simulink model "lab5"  (R2014b)
settings: Solver=ode45  SolverMode=SingleTasking  StartTime=0.0  StopTime=10  RelTol=1e-3
libraries: truetime x1
settings Model: Creator=peterfj  LastModifiedBy=andfro
settings OptimizationCC: BlockReduction=off  BooleanDataType=off  UseDivisionForNetSlopeComputation=off  SimCompilerOptimization=off
settings DebuggingCC: SaveWithParameterizedLinksMsg=none  UnderspecifiedInitializationDetection=Classic  MergeDetectMultiDrivingBlocksExec=none  SignalResolutionControl=TryResolveAllWithWarning  SolverPrmCheckMsg=none  FrameProcessingCompatibilityMsg=error  AllowSymbolicDim=off
settings HardwareCC: TargetUnknown=on
settings RTWCC: RTWCompilerOptimization=off
settings ConfigComp: CovMetricSettings=dw  CovHtmlReporting=on  CovSaveCumulativeToWorkspaceVar=on  CovSaveSingleToWorkspaceVar=on  CovModelRefEnable=Off  CovExternalEMLEnable=off  CovSFcnEnable=off

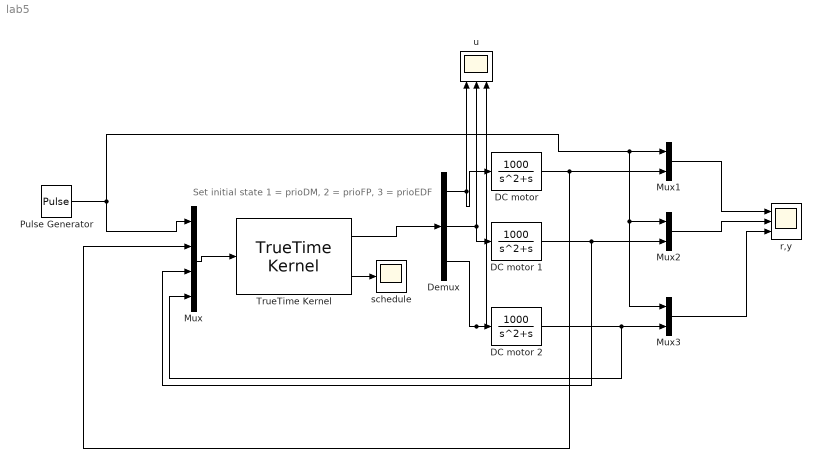
== system lab5 ==
  note: Set initial state 1 = prioDM, 2 = prioFP, 3 = prioEDF
  "DC motor " : TransferFcn  Numerator=[1000]  Denominator=[1 1 0]
  DC motor 1 : TransferFcn  Numerator=[1000]  Denominator=[1 1 0]
  DC motor 2 : TransferFcn  Numerator=[1000]  Denominator=[1 1 0]
  Demux : Demux  Outputs=3
  Mux : Mux
  Mux1 : Mux  Inputs=2
  Mux2 : Mux  Inputs=2
  Mux3 : Mux  Inputs=2
  Pulse Generator : DiscretePulseGenerator  PulseType=Time based  Amplitude=2  Period=1  PulseWidth=50  PhaseDelay=0.1  SampleTime=0.005
  TrueTime Kernel : truetime/TrueTime Kernel  sfun=node_init_3  args=1  ninputsoutputs=[4 3]  ntriggers=0  trigtype=falling  nwnodenbr=[]  clockoffsetdrift=[0 0]  schedoutput=on  battery=off  poweroutput=off
  r,y : Scope  NumInputPorts=3
      settings: ShowLegends=on  YMin=-0.36389~-5~-5  YMax=2.36389~5~5
  schedule : Scope
      settings: TimeRange=5  YMin=1  YMax=1.5
  u : Scope  NumInputPorts=3
      settings: ShowLegends=on  YMin=-1.34892~-5~-5  YMax=1.34892~5~5  SaveName=ScopeData2
  wires:
  Mux/1 -> TrueTime Kernel/1
  TrueTime Kernel/2 -> schedule/1
  Pulse Generator/1 -> Mux/1, Mux3/1, Mux2/1, Mux1/1
  "DC motor "/1 -> Mux1/2, Mux/2
  DC motor 1/1 -> Mux/3, Mux2/2
  DC motor 2/1 -> Mux/4, Mux3/2
  Mux1/1 -> r,y/1
  Mux2/1 -> r,y/2
  Mux3/1 -> r,y/3
  TrueTime Kernel/1 -> Demux/1
  Demux/1 -> "DC motor "/1, u/1
  Demux/2 -> DC motor 1/1, u/2
  Demux/3 -> u/3, DC motor 2/1
